simulink model "fading"  (Simulink 4.00)
settings: Solver=ode45  StartTime=0.0  StopTime=.6  RelTol=1e-3
undefined symbols (not defined in the file): j, slcm
libraries: commchan2 x2, dspsrcs3 x1
settings Model: LastModifiedBy=agaltman  BlockReductionOpt=off

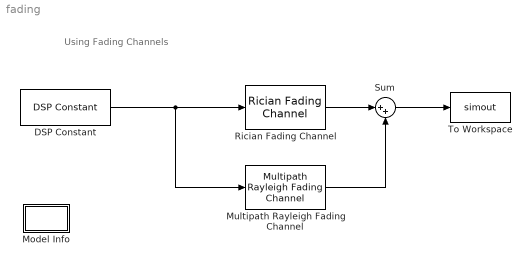
== system fading ==
  note: Using Fading Channels
  DSP Constant : dspsrcs3/DSP Constant  Value=j*ones(10000,1)  InterpretAs1D=off  SampleMode=Discrete  Ts=.01  FramebasedOutput=on
  Model Info : Subsystem  LoadFcn=slcm LoadBlock;  InitFcn=slcm('UpdateAllCMBlocksInThisModelInit')  mask(CMBlock){InitialSaveTempField=, InitialBlockCM=none, BlockCM=none, Frame=on, SaveTempField=, DisplayStringWithTags=Info, MaskDisplayString=Info, HorizontalTextAlignment=Center, LeftAlignmentValue=0.5, SourceBlockDiagram=fading, TagMaxNumber=20, CMTag1=, CMTag2=, CMTag3=, CMTag4=, CMTag5=, CMTag6=, CMTag7=, CMTag8=, CMTag9=, CMTag10=, CMTag11=, CMTag12=, CMTag13=, CMTag14=, CMTag15=, CMTag16=, CMTag17=, CMTag18=, CMTag19=, CMTag20=}
      mask help: This block allows revision control information to be displayed within the model.
      settings: CopyFcn=slcm CopyBlock;  DeleteFcn=slcm Cancel;  PostSaveFcn=slcm('UpdateAllCMBlocksInThisModel')  NameChangeFcn=slcm Rename;  OpenFcn=commdemohelp;  RTWFcnNameOpts=Auto  RTWFileNameOpts=Auto
      mask Display: text(str2num(LeftAlignmentValue), 0.5, MaskDisplayString, 'HorizontalAlignment', HorizontalTextAlignment)
  Multipath Rayleigh Fading Channel : commchan2/Multipath Rayleigh Fading Channel  Fd=40  simTs=1e-6  delayVec=[0 2e-6 3e-6]  gainVecdB=[0 -3 1]  normGain=on  Seed=12345
  Rician Fading Channel : commchan2/Rician Fading Channel  K=1  Fd=40  simTs=1e-6  delayVec=0  gainVecdB=0  Seed=12345
  Sum : Sum  Inputs=|++  SaturateOnIntegerOverflow=on
  To Workspace : ToWorkspace  VariableName=simout  SampleTime=-1  SaveFormat=Array
  wires:
  DSP Constant/1 -> Rician Fading Channel/1, Multipath Rayleigh Fading Channel/1
  Sum/1 -> To Workspace/1
  Rician Fading Channel/1 -> Sum/1
  Multipath Rayleigh Fading Channel/1 -> Sum/2

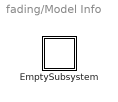
== system fading/Model Info ==
  EmptySubsystem : Subsystem
      settings: RTWFcnNameOpts=Auto  RTWFileNameOpts=Auto

== system fading/Model Info/EmptySubsystem ==
